simulink model "term"  (R2020a)
settings: Solver=VariableStepAuto  StartTime=0.0  StopTime=5  RelTol=1e-3
values from neighbouring files (symbols this model uses):
  F = [0      1              0           0 ... (first row only)    [Pedulum_Cart.m]
  Faa = [0 0;0 2.6727]    [Pedulum_Cart.m]
  Fab = [ 1 0 ;-0.1818 0]    [Pedulum_Cart.m]
  Fba = [ 0 0; 0 31.1818]    [Pedulum_Cart.m]
  Fbb = [ 0 1 ... (first row only)    [Pedulum_Cart.m]
  G = [     0 ... (first row only)    [Pedulum_Cart.m]
  Ga = [0; 0]    [Pedulum_Cart.m]
  Gb = [ 1.8182 ; 4.5455]    [Pedulum_Cart.m]
  H = [1 0 0 0 ... (first row only)    [Pedulum_Cart.m]
  K_itg0 = [K_itg(1)]    [Pedulum_Cart.m]
  K_itg1 = [K_itg(2) K_itg(3) K_itg(4) K_itg(5) ]    [Pedulum_Cart.m]
  K_lqr = lqr(F,G,Q,R)    [Pedulum_Cart.m]
  L = place(F',H',P)'    [Pedulum_Cart.m]
  L_re = Lt_re'    [Pedulum_Cart.m]
  Nbar = rscale(sys_ss,K_lqr)    [Pedulum_Cart.m]    (also in rscale.m = Nu + K*Nx)
libraries: simulink x1
settings Model: Creator=Robpang  LastModifiedBy=RoboticsAndAI

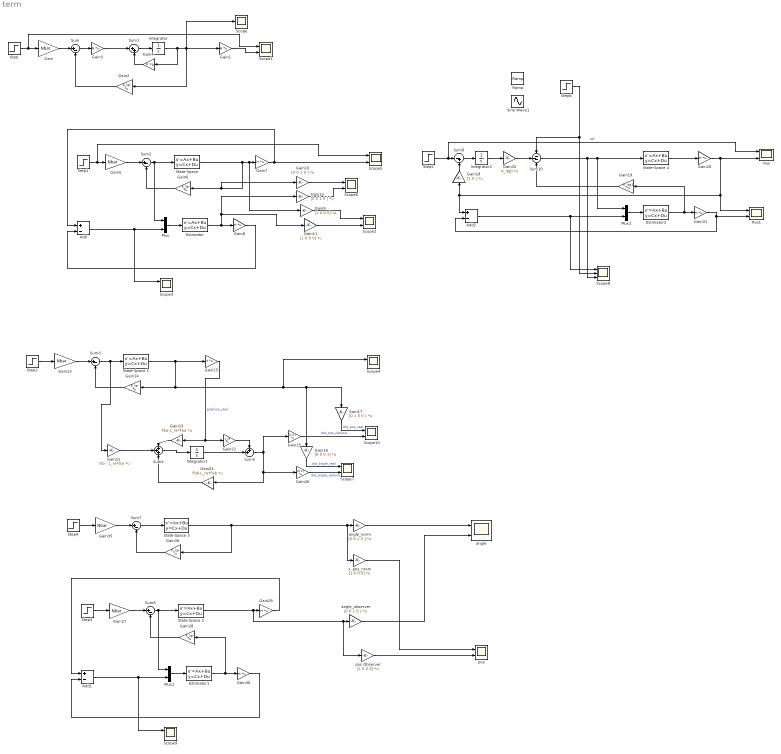
== system term ==
  " Estimator" : StateSpace  A=F  B=[G L]  C=eye(4)  D=zeros(4,3)  InitialCondition=[5 0 1 0]
  " Estimator1" : StateSpace  A=F  B=[G L]  C=eye(4)  D=zeros(4,3)  InitialCondition=[0 0 0 0]
  " Estimator2" : StateSpace  A=F  B=[G L]  C=eye(4)  D=zeros(4,3)  InitialCondition=[0 0 0 0]
  " State-Space " : StateSpace  A=F  B=G  C=eye(4)  D=zeros(4,1)  InitialCondition=[0 0 0 0]
  " State-Space 1" : StateSpace  A=F  B=G  C=eye(4)  D=zeros(4,1)  InitialCondition=[0 0 0 0]
  " State-Space 2" : StateSpace  A=F  B=G  C=eye(4)  D=zeros(4,1)  InitialCondition=[1 0 0 0]
  " State-Space 3" : StateSpace  A=F  B=G  C=eye(4)  D=zeros(4,1)  InitialCondition=[0 0 0 0]
  " State-Space 4" : StateSpace  A=F  B=G  C=[1 0 0 0; 0 1 0 0; 0 0 1 0; 0 0 1 0]  D=zeros(4,1)  InitialCondition=[0 0 0 0]
  Add : Sum  Inputs=+-
  Add1 : Sum  Inputs=+-
  Add2 : Sum  Inputs=+-
  Gain{,5,13,27,35} (5 alike) : Gain  Gain=Nbar
  Gain{1,7..8,15,20,29..31} (8 alike) : Gain  Gain=H  Multiplication=Matrix(K*u)
  Gain10 : Gain  Gain=[0 0 1 0 ]  Multiplication=Matrix(K*u)
  Gain11 : Gain  Gain=[1 0 0 0]  Multiplication=Matrix(K*u)
  Gain12 : Gain  Gain=[0 0 1 0 ]  Multiplication=Matrix(K*u)
  Gain{2,6,14,28,36} (5 alike) : Gain  Gain=K_lqr  Multiplication=Matrix(K*u)
  Gain16 : Gain  Gain=[0 0 0 1]  Multiplication=Matrix(K*u)
  Gain17 : Gain  Gain=[0 1 0 0 ]  Multiplication=Matrix(K*u)
  Gain18 : Gain  Gain=[1 0 ]  Multiplication=Matrix(K*u)
  Gain19 : Gain  Gain=K_itg1  Multiplication=Matrix(K*u)
  Gain21 : Gain  Gain=Gb - L_re*Ga  Multiplication=Matrix(K*u)
  Gain22 : Gain  Gain=L_re  Multiplication=Matrix(K*u)
  Gain23 : Gain  Gain=Fba-L_re*Faa  Multiplication=Matrix(K*u)
  Gain24 : Gain  Gain=Fbb-L_re*Fab  Multiplication=Matrix(K*u)
  Gain25 : Gain  Gain=[1 0 ]  Multiplication=Matrix(K*u)
  Gain26 : Gain  Gain=[0 1]  Multiplication=Matrix(K*u)
  Gain3 : Gain  Gain=G  Multiplication=Matrix(K*u)
  Gain32 : Gain  Gain=K_itg0  Multiplication=Matrix(K*u)
  Gain4 : Gain  Gain=F  Multiplication=Matrix(K*u)
  Gain9 : Gain  Gain=[1 0 0 0]  Multiplication=Matrix(K*u)
  Integrator : Integrator
  Integrator1 : Integrator
  Integrator2 : Integrator
  Mux : Mux  Inputs=2
  Mux1 : Mux  Inputs=2
  Mux2 : Mux  Inputs=2
  Pos : Scope  NumInputPorts=2
  Pos1 : Scope  NumInputPorts=2
  Ramp : simulink/Sources/Ramp  slope=50  start=1  InitialOutput=0
  Scope : Scope
  Scope{1..7,9..10} (9 alike) : Scope  NumInputPorts=2
  Scope8 : Scope  NumInputPorts=3
  Sine Wave1 : Sin  Amplitude=50  Frequency=10  SampleTime=0
  Step : Step  Time=0  After=[1 0 0 0]  SampleTime=0
  Step{1..5} (5 alike) : Step  Time=0  After=5  SampleTime=0
  Step6 : Step  After=50  SampleTime=0
  Sum{,2..3,6..7} (5 alike) : Sum  Inputs=|+-
  Sum1 : Sum  Inputs=|++
  Sum10 : Sum  Inputs=---
  Sum4 : Sum  Inputs=+++
  Sum5 : Sum  Inputs=++|
  Sum9 : Sum  Inputs=|-+
  angle : Scope  NumInputPorts=2
  angle_norm : Gain  Gain=[0 0 1 0 ]  Multiplication=Matrix(K*u)
  angle_observer : Gain  Gain=[0 0 1 0 ]  Multiplication=Matrix(K*u)
  pos : Scope  NumInputPorts=2
  pos Observer : Gain  Gain=[1 0 0 0]  Multiplication=Matrix(K*u)
  x_pos_nrom : Gain  Gain=[1 0 0 0]  Multiplication=Matrix(K*u)
  wires:
  Gain/1 -> Sum/1
  Sum/1 -> Gain3/1
  Gain1/1 -> Scope1/2
  Integrator/1 -> Gain4/1, Gain2/1, Scope/1, Gain1/1
  Gain2/1 -> Sum/2
  Gain3/1 -> Sum1/1
  Sum1/1 -> Integrator/1
  Gain4/1 -> Sum1/2
  Step/1 -> Scope1/1, Gain/1
  Step1/1 -> Scope5/1, Gain5/1
  " State-Space "/1 -> Gain10/1, Gain6/1, Gain9/1, Gain7/1
  Gain6/1 -> Sum2/2
  Gain5/1 -> Sum2/1
  Sum2/1 -> Mux/1, " State-Space "/1
  Gain7/1 -> Add/1, Scope5/2
  Add/1 -> Scope3/1, Mux/2
  Mux/1 -> " Estimator"/1
  " Estimator"/1 -> Gain11/1, Gain12/1, Gain8/1
  Gain8/1 -> Add/2
  Gain9/1 -> Scope2/1
  Gain11/1 -> Scope2/2
  Gain10/1 -> Scope6/1
  Gain12/1 -> Scope6/2
  Sum4/1 -> Integrator1/1
  Gain22/1 -> Sum5/1
  Gain23/1 -> Sum4/1
  Gain14/1 -> Sum3/2
  Gain24/1 -> Sum4/3
  Gain15/1 -> Gain22/1, Gain23/1  "position_real"
  Sum5/1 -> Gain25/1, Gain26/1, Gain24/1
  Gain25/1 -> Scope10/2  "dot_pos_reduce"
  " State-Space 1"/1 -> Scope4/1, Gain16/1, Gain17/1, Gain14/1, Gain15/1
  Gain21/1 -> Sum4/2
  Integrator1/1 -> Sum5/2
  Sum3/1 -> Gain21/1, " State-Space 1"/1
  Gain13/1 -> Sum3/1
  Step2/1 -> Gain13/1
  Gain16/1 -> Scope7/1  "dot_angle_real"
  Gain17/1 -> Scope10/1  "dot_pos_real"
  Gain26/1 -> Scope7/2  "dot_angle_reduce"
  angle_observer/1 -> angle/2
  angle_norm/1 -> angle/1
  Gain30/1 -> Add1/2
  Gain27/1 -> Sum6/1
  Mux1/1 -> " Estimator1"/1
  Gain29/1 -> Add1/1
  Add1/1 -> Scope9/1, Mux1/2
  x_pos_nrom/1 -> pos/1
  pos Observer/1 -> pos/2
  Step3/1 -> Gain27/1
  " State-Space 2"/1 -> pos Observer/1, angle_observer/1, Gain29/1
  Sum6/1 -> Mux1/1, " State-Space 2"/1
  Gain28/1 -> Sum6/2
  " Estimator1"/1 -> Gain28/1, Gain30/1
  Gain36/1 -> Sum7/2
  " State-Space 3"/1 -> Gain36/1, x_pos_nrom/1, angle_norm/1
  Sum7/1 -> " State-Space 3"/1
  Step4/1 -> Gain35/1
  Gain35/1 -> Sum7/1
  Gain31/1 -> Pos1/2, Add2/2
  Mux2/1 -> " Estimator2"/1
  " Estimator2"/1 -> Gain19/1, Gain31/1
  Gain19/1 -> Sum10/3
  " State-Space 4"/1 -> Gain20/1
  Gain20/1 -> Pos/2, Pos1/1, Gain18/1, Add2/1
  Sum10/1 -> Mux2/1, " State-Space 4"/1, Scope8/3
  Add2/1 -> Scope8/1, Mux2/2
  Sum9/1 -> Integrator2/1
  Integrator2/1 -> Gain32/1
  Step5/1 -> Pos/1, Sum9/1  "ref"
  Gain32/1 -> Sum10/2
  Step6/1 -> Sum10/1, Scope8/2
  Gain18/1 -> Sum9/2
